simulink model "tm01"  (Simulink 8.1)
settings: Solver=ode45  StartTime=0.0  StopTime=10000  RelTol=1e-3
settings Model: Creator=my88899  LastModifiedBy=my88899
settings DataIOCC: SignalLoggingSaveFormat=Dataset
settings OptimizationCC: ExpressionDepthLimit=128
settings DebuggingCC: FcnCallInpInsideContextMsg=EnableAllAsError
settings GRTTargetCC: CombineOutputUpdateFcns=on  GRTInterface=off

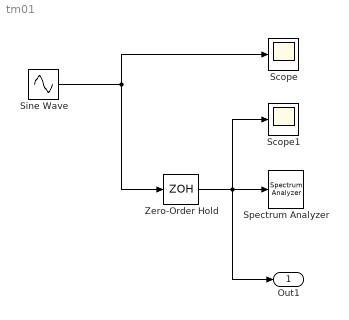
== system tm01 ==
  Scope : Scope
      settings: TimeRange=5000  YMin=-2  YMax=2
  Scope1 : Scope
      settings: TimeRange=5000  YMin=-2  YMax=2
  Sine Wave : Sin  Amplitude=2  Frequency=1000  SampleTime=0
  Spectrum Analyzer : SpectrumAnalyzer
      settings: CopyFcn=scopeextensions.ScopeBlock.callback(gcbh, 'onBlockCopy', gcbh);  DeleteFcn=scopeextensions.ScopeBlock.callback(gcbh, 'onBlockDelete');  PreSaveFcn=scopeextensions.ScopeBlock.callback(gcbh, 'onModelSave');  NameChangeFcn=scopeextensions.ScopeBlock.callback(gcbh, 'onBlockRename');  CloseFcn=scopeextensions.ScopeBlock.callback(gcbh, 'onBlockClose');  PreDeleteFcn=scopeextensions.ScopeBlock.callback(gcbh, 'onBlockPreDelete');
  Zero-Order Hold : ZeroOrderHold
  Out1 : Outport
  wires:
  Sine Wave/1 -> Zero-Order Hold/1, Scope/1
  Zero-Order Hold/1 -> Out1/1, Scope1/1, Spectrum Analyzer/1
